simulink model "sldemo_mdlref_heater"  (Simulink 7.6)
settings: Solver=ode3  SolverMode=SingleTasking  StartTime=0.0  StopTime=2*24*60*60  FixedStep=60  RelTol=1e-3  AbsTol=1e-6
model workspace (MAT data in the model file):
  ha = 304636.2
  Mdot : num (value not decoded)
settings Model: Creator=The MathWorks Inc.  ExtModeAutoUpdateStatusClock=off
settings DataIOCC: ExternalInput=[]  InitialState=[]  LimitDataPoints=off  SaveOutput=off  SaveTime=off
settings OptimizationCC: BlockReduction=off  BooleanDataType=off  InlineParams=on  InlineInvariantSignals=on  InitFltsAndDblsToZero=on
settings DebuggingCC: SaveWithParameterizedLinksMsg=none  CheckExecutionContextPreStartOutputMsg=on  CheckExecutionContextRuntimeOutputMsg=on  SolverPrmCheckMsg=none  MultiTaskDSMMsg=warning  MultiTaskCondExecSysMsg=none  SigSpecEnsureSampleTimeMsg=none  IntegerOverflowMsg=none
settings RTWCC: IncludeERTFirstTime=on
settings CodeAppCC: MaxIdLength=100
settings GRTTargetCC: TargetFcnLib=ansi_tfl_tmw.mat

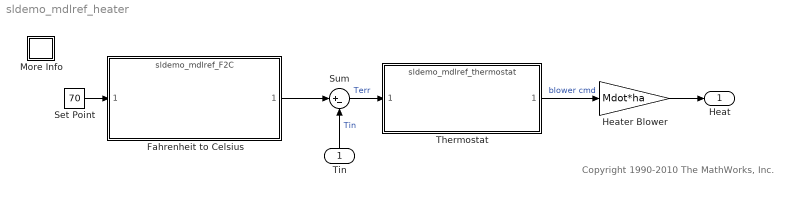
== system sldemo_mdlref_heater ==
  note: Copyright 1990-2010 The MathWorks, Inc.
  Tin : Inport  OutDataTypeStr=double  PortDimensions=1  SampleTime=0
  Fahrenheit to Celsius : ModelReference  ModelNameDialog=sldemo_mdlref_F2C  SimulationMode=Normal  ModelReferenceVersion=1.15  CopyOfModelName=sldemo_mdlref_F2C
  Heater Blower : Gain  Gain=Mdot*ha  SaturateOnIntegerOverflow=on  OutDataTypeStr=Inherit: Same as input  ParamDataTypeStr=Inherit: Same as input
  More Info : Subsystem
      settings: OpenFcn=showdemo('sldemo_mdlref_depgraph')
      mask Display: disp('?')
  Set Point : Constant  Value=70
  Sum : Sum  Inputs=|+-  SaturateOnIntegerOverflow=on  InputSameDT=on  OutDataTypeStr=Inherit: Same as first input
  Thermostat : ModelReference  ModelNameDialog=sldemo_mdlref_thermostat  SimulationMode=Accelerator  ModelReferenceVersion=1.13  CopyOfModelName=sldemo_mdlref_thermostat
  Heat : Outport
  wires:
  Heater Blower/1 -> Heat/1
  Thermostat/1 -> Heater Blower/1  "blower cmd"
  Tin/1 -> Sum/2  "Tin"
  Sum/1 -> Thermostat/1  "Terr"
  Fahrenheit to Celsius/1 -> Sum/1
  Set Point/1 -> Fahrenheit to Celsius/1

== system sldemo_mdlref_heater/More Info ==
